simulink model "project_final"  (R2022b)
settings: Solver=VariableStepAuto  StartTime=0.0  StopTime=20  RelTol=1e-3
values from neighbouring files (symbols this model uses):
  A = [0 0 0 1 0 0 0 0 0 0 0 0;     0 0 0 0 1 0 0 0 0 0 0 0;     0 0 0 0 0 1 0 0 0 0 0 0;     0 0 0 0 0 0 0 -g 0 0 0 0;     0 0 0 0 0 0 g 0 0 0 0 0;     0 0 0 0 0 0 0 0 0 0 0 0;     0 0 0 0 0 0 0 0 0 1 0 0;     0 0 0 0 0 0 0 0 0 0 1 0;     0 0 0 0 0 0 0 0 0 0 0 1;     0 0 0 0 0 0 0 0 0 0 0 0;     0 0 0 0 0 0 0 0 0 0 0 0;     0 0 0 0 0 0 0 0 0 0 0 0]    [project_final.m]
  Ax = 0.0    (= 0)    [project_final.m]
  Ay = 0.0    (= 0)    [project_final.m]
  Az = 0.0    (= 0)    [project_final.m]
  B = [0 0 0 0;     0 0 0 0;     0 0 0 0;     0 0 0 0;     0 0 0 0;     1/m 0 0 0;     0 0 0 0;     0 0 0 0;     0 0 0 0;     0 1/Ixx 0 0;     0 0 1/Iyy 0;     0 0 0 1/Izz;]    [project_final.m]
  C = [1 0 0 0 0 0 0 0 0 0 0 0;      0 1 0 0 0 0 0 0 0 0 0 0;      0 0 1 0 0 0 0 0 0 0 0 0;      0 0 0 0 0 0 1 0 0 0 0 0;      0 0 0 0 0 0 0 1 0 0 0 0;      0 0 0 0 0 0 0 0 1 0 0 0;]    [project_final.m]
  D = zeros(6,4)    [project_final.m]
  g = 9.81    [project_final.m]
  Ixx = 0.00963    [project_final.m]
  Iyy = 0.00963    [project_final.m]
  Izz = 0.019    [project_final.m]
  Jr = 5.225e-5    (= 5.225e-05)    [project_final.m]
  l = 0.24    [project_final.m]
  m = 0.82    [project_final.m]
undefined symbols (not defined in the file or in its folder): K_n, K_o, sysK
libraries: simulink x5, simulink_extras x4, visionsinks x2, sim3dcameralib x2, sim3dlib x2, uavsim3dlib x2
settings Model: Creator=isa  LastModifiedBy=Abdullah Ak
settings SolverCC: ZeroCrossAlgorithm=Adaptive
settings DataIOCC: ReturnWorkspaceOutputs=off
settings DebuggingCC: MaskedZcDiagnostic=none  IgnoredZcDiagnostic=none

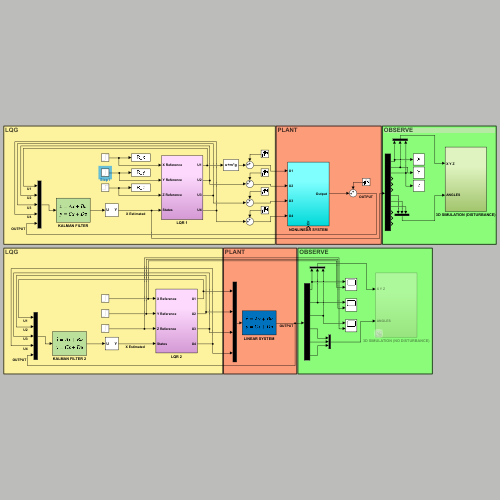
[thumbnail: Simulink's stored preview of the top-level diagram]
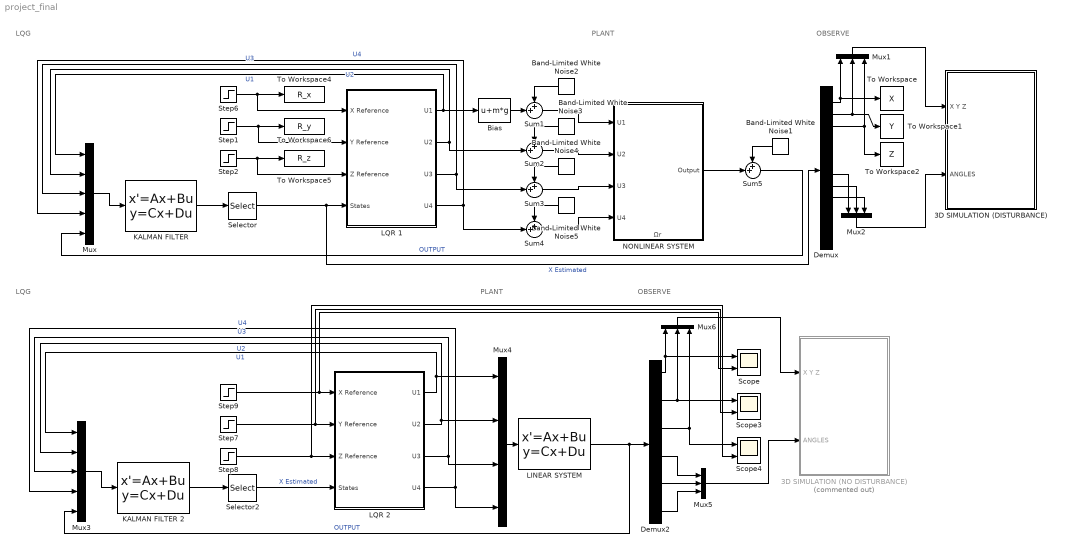
== system project_final ==
  note: OBSERVE
  note: OBSERVE
  note: PLANT
  note: LQG
  note: LQG
  note: PLANT
  3D SIMULATION (DISTURBANCE) : Subsystem
  3D SIMULATION (NO DISTURBANCE) : Subsystem  Commented=on
  Band-Limited White Noise{1..5} (5 alike) : simulink/Sources/Band-Limited White Noise  Cov=[0.0001]  Ts=0.1  seed=[23341]
  Bias : Bias  Bias=m*g  SaturateOnIntegerOverflow=off
  Demux : Demux  Outputs=12
  Demux2 : Demux  Outputs=6
  KALMAN FILTER : StateSpace  A=sysK.A  B=sysK.B  C=sysK.C  D=sysK.D  InitialCondition=0
  KALMAN FILTER 2 : StateSpace  A=sysK.A  B=sysK.B  C=sysK.C  D=sysK.D  InitialCondition=0
  LINEAR SYSTEM : StateSpace  A=A  B=B  C=C  D=D  InitialCondition=0
  LQR 1 : Subsystem
  LQR 2 : Subsystem
  Mux : Mux  Inputs=5
  Mux{1..2,5..6} (4 alike) : Mux  Inputs=3
  Mux3 : Mux  Inputs=5
  Mux4 : Mux
  NONLINEAR SYSTEM : Subsystem
      settings: PortSchema="{\"entries\":[{\"content\":{\"sides\":[{\"content\":{\"connectorIds\":[\"In1\",\"In2\",\"In3\",\"In4\"]},\"type\":\"ConnectorPlacement.EquallySpacedRectSide\",\"uuid\":\"a5503451-5a23-4017-b645-9eb3d3f2dd65\"},{\"content\":{\"connectorIds\":[\"Out1\"],\"side\":\"RIGHT\"},\"type\":\"ConnectorPlacement.EquallySpacedRectSide\",\"uuid\":\"5f9284f0-a452-4177-bce3-aee519bf0d63\"},{\"content\":{\"side\":\"TOP\"},\"type\":\"ConnectorPlacement.EquallySpacedRectSide\",\"uuid\":\"8bc8bc99-887e-4f77-aaa8-21d509049f1f\"},{\"content\":{\"connectorIds\":[\"In5\"],\"side\":\"BOTTOM\"},\"type\":\"ConnectorPlacement.EquallySpacedRectSide\",\"uuid\":\"ae093331-e5e5-4be8-9937-2af24c161ac0\"}]},\"type\":\"ConnectorPlacement.EquallySpacedConnector\",\"uuid\":\"9aea3e95-818c-4bf6-8240-35747b8e2613\"}],\"packageUris\":[\"http://schema.mathworks.com/mf0/Connector/R2020b\"],\"version\":\"1.0\"}"
  Scope : Scope  NumInputPorts=2
  Scope3 : Scope  NumInputPorts=2
  Scope4 : Scope  NumInputPorts=2
  Selector : Selector  InputPortWidth=18  IndexOptions=Index vector (dialog)  Indices=[7:18]  OutputSizes=1
  Selector2 : Selector  InputPortWidth=18  IndexOptions=Index vector (dialog)  Indices=[7:18]  OutputSizes=1
  Step1 : Step  Time=5  After=25  SampleTime=0
  Step2 : Step  After=31  SampleTime=0
  Step6 : Step  Time=10  After=31  SampleTime=0
  Step7 : Step  Time=5  After=8  SampleTime=0
  Step8 : Step  After=10  SampleTime=0
  Step9 : Step  Time=10  After=8  SampleTime=0
  Sum{1..5} (5 alike) : Sum  Inputs=++|
  To Workspace : ToWorkspace  VariableName=X  SaveFormat=Timeseries  SampleTime=-1
  To Workspace1 : ToWorkspace  VariableName=Y  SaveFormat=Timeseries  SampleTime=-1
  To Workspace2 : ToWorkspace  VariableName=Z  SaveFormat=Timeseries  SampleTime=-1
  To Workspace4 : ToWorkspace  VariableName=R_x  SaveFormat=Timeseries  SampleTime=-1
  To Workspace5 : ToWorkspace  VariableName=R_z  SaveFormat=Timeseries  SampleTime=-1
  To Workspace6 : ToWorkspace  VariableName=R_y  SaveFormat=Timeseries  SampleTime=-1
  wires:
  LQR 1/1(U1) -> Bias/1, Mux/1  "U1"
  Bias/1 -> Sum1/2
  LQR 1/2(U2) -> Sum2/2, Mux/2  "U2"
  LQR 1/3(U3) -> Sum3/2, Mux/3  "U3"
  LQR 1/4(U4) -> Sum4/2, Mux/4  "U4"
  KALMAN FILTER/1 -> Selector/1
  Selector/1 -> LQR 1/4(States), Demux/1  "X Estimated"
  Mux/1 -> KALMAN FILTER/1
  Sum5/1 -> Mux/5  "OUTPUT"
  Step1/1 -> LQR 1/2(Y Reference), To Workspace6/1
  Step6/1 -> To Workspace4/1, LQR 1/1(X Reference)
  Step2/1 -> LQR 1/3(Z Reference), To Workspace5/1
  Demux/3 -> To Workspace2/1, Mux1/3
  Demux/1 -> Mux1/1, To Workspace/1
  Demux/2 -> To Workspace1/1, Mux1/2
  Sum1/1 -> NONLINEAR SYSTEM/1(U1)
  Sum2/1 -> NONLINEAR SYSTEM/2(U2)
  Sum3/1 -> NONLINEAR SYSTEM/3(U3)
  Sum4/1 -> NONLINEAR SYSTEM/4(U4)
  NONLINEAR SYSTEM/1("Output ") -> Sum5/2
  Band-Limited White Noise1/1 -> Sum5/1
  Band-Limited White Noise2/1 -> Sum1/1
  Band-Limited White Noise3/1 -> Sum2/1
  Band-Limited White Noise4/1 -> Sum3/1
  Band-Limited White Noise5/1 -> Sum4/1
  Demux2/2 -> Scope3/1, Mux6/2
  Demux2/3 -> Scope4/1, Mux6/3
  Step8/1 -> LQR 2/3(Z Reference), Scope4/2
  Step9/1 -> LQR 2/1(X Reference), Scope/2
  Step7/1 -> LQR 2/2(Y Reference), Scope3/2
  LINEAR SYSTEM/1 -> Mux3/5, Demux2/1  "OUTPUT"
  Mux3/1 -> KALMAN FILTER 2/1
  Selector2/1 -> LQR 2/4(States)  "X Estimated"
  KALMAN FILTER 2/1 -> Selector2/1
  LQR 2/4(U4) -> Mux4/4, Mux3/4  "U4"
  LQR 2/3(U3) -> Mux4/3, Mux3/3  "U3"
  LQR 2/2(U2) -> Mux4/2, Mux3/2  "U2"
  LQR 2/1(U1) -> Mux3/1, Mux4/1  "U1"
  Mux4/1 -> LINEAR SYSTEM/1
  Demux2/1 -> Scope/1, Mux6/1
  Demux2/4 -> Mux5/1
  Demux2/5 -> Mux5/2
  Demux2/6 -> Mux5/3
  Mux6/1 -> 3D SIMULATION (NO DISTURBANCE)/1(X Y Z)
  Mux5/1 -> 3D SIMULATION (NO DISTURBANCE)/2(ANGLES)
  Mux1/1 -> 3D SIMULATION (DISTURBANCE)/1(X Y Z)
  Mux2/1 -> 3D SIMULATION (DISTURBANCE)/2(ANGLES)
  Demux/8 -> Mux2/2
  Demux/9 -> Mux2/3
  Demux/7 -> Mux2/1

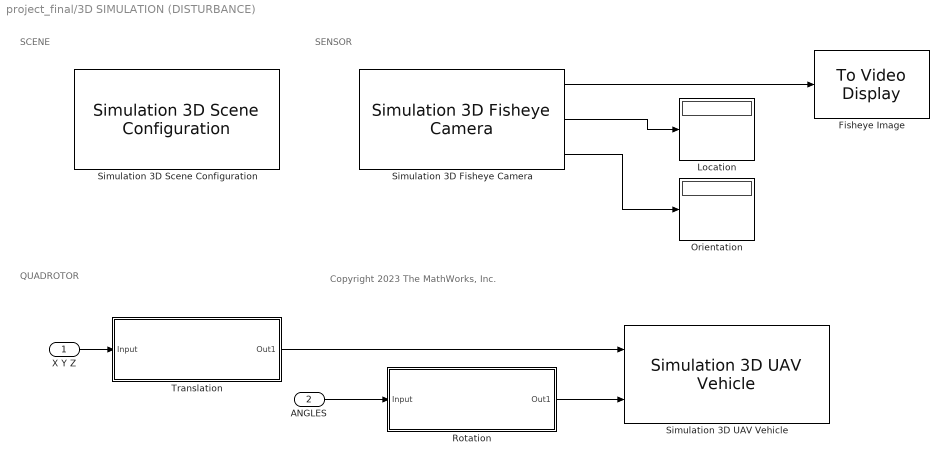
== system project_final/3D SIMULATION (DISTURBANCE) ==
  note: SCENE
  note: QUADROTOR
  note: SENSOR
  note: Copyright 2023 The MathWorks, Inc.
  X Y Z : Inport
  ANGLES : Inport  Port=2
  Fisheye Image : visionsinks/To Video Display  windowSizeMode=Normal  openAtMdlStart=on  fullScreen=off  videoWindowX=2625  videoWindowY=376  saveWindowSize=off  videoWindowWidth=640  videoWindowHeight=640  inputColorFormat=RGB  inputType=Obsolete  imagePorts=One multidimensional signal  OutputDevice=On-screen video monitor  dataOrg=Column-major  isWindowOpen=off
  Location : Display
  Orientation : Display
  Rotation : Subsystem
  Simulation 3D Fisheye Camera : sim3dcameralib/Simulation 3D Fisheye Camera  Priority=1  sensorTag=Sim3dSensor3  sensorId=3  sensorName=Sim3dSensor3  vehTagList={'Q_D';'Scene Origin'}  vehTag=Q_D  mountLoc=Origin  offsetFlag=on  tmountOffset=[0.1, 0, 0]  extTmount=off  rmountOffset=[0, 0, 0]  extRmount=off  OpticalCenter=[640, 360]  ImageSize=[720, 1280]  RadialDistortion=[320, -0.0005, 0, 0]  StretchMatrix=[1, 0; 0, 1]  TransformOutportEnabled=on  SampleTime=-1  mountPoint=[0.1 0 0]  mountOrientation=[0 0 0]  aMode=4  ID=3
  Simulation 3D Scene Configuration : sim3dlib/Simulation 3D Scene Configuration  Priority=0  ProjectFormat=Default Scenes  SceneDesc=US city block  ProjectName=D:\Programlar\MATLAB\R2022B\toolbox\shared\sim3d_projects\automotive_project\UE4\WindowsNoEditor\VehicleSimulation.exe  ScenePath=/Game/Maps/USCityBlock  EnableOpenDRIVE=off  vehTagList={'Q_D';'Scene Origin'}  vehTag=Q_D  OpVisEn=off  Ts=0.3  EnableWindow=on  EnableRemoteAccess=off  EnableWeather=off  SunAltitude=40.0  SunAzimuth=90  clouds=10  wind=0.0  fog=20.0  rain=30  EnableGeospatial=off  OriginHeight=200  OriginLatitude=40.744652  OriginLongitude=-73.988864  MapStyle=Aerial  AdditionalAssetIDs=[]  UseAdvancedSunSky=off  SolarTime=11  TimeZone=-5  Day=21  Month=9  Year=2022  UseDaylightSavingTime=on  DSTStartDay=10  DSTStartMonth=3  DSTEndDay=3  DSTEndMonth=11  DSTSwitchHour=2  sensorTag=MainCamera3  sensorId=3  sensorName=MainCamera3  mountLoc=Origin  offsetFlag=off  tmountOffset=[0, 0, 0]  rmountOffset=[0, 0, 0]  HorizontalResolution=1280  VerticalResolution=720  HorizontalFOV=60  mountPoint=[0 0 0]  mountOrientation=[0 0 0]  aMode=4  ID=3  GeoTrigger=Inactive
  Simulation 3D UAV Vehicle : uavsim3dlib/Simulation 3D UAV Vehicle  Mesh=Quadrotor  MeshPath=/MathWorksUAVContent/UAVs/HexaRotorUAV/HexaRotor.HexaRotor  Color=Black  ActorName=Q_D  InitialTranslation=[0 5 1.5]  InitialRotation=[0 0 0]  SampleTime=-1  ActorType=SimulinkVehicle  ID=C  aMode=4  ActorTag=Q_D
  Translation : Subsystem
  wires:
  Simulation 3D Fisheye Camera/1 -> Fisheye Image/1
  Translation/1(Out1) -> Simulation 3D UAV Vehicle/1
  Simulation 3D Fisheye Camera/3 -> Orientation/1
  X Y Z/1 -> Translation/1(Input)
  ANGLES/1 -> Rotation/1(Input)
  Rotation/1(Out1) -> Simulation 3D UAV Vehicle/2
  Simulation 3D Fisheye Camera/2 -> Location/1

== system project_final/3D SIMULATION (NO DISTURBANCE) ==
  note: SENSOR
  note: QUADROTOR
  note: SCENE
  X Y Z : Inport
  ANGLES : Inport  Port=2
  Fisheye Image : visionsinks/To Video Display  windowSizeMode=Normal  openAtMdlStart=on  fullScreen=off  videoWindowX=2625  videoWindowY=376  saveWindowSize=off  videoWindowWidth=640  videoWindowHeight=640  inputColorFormat=RGB  inputType=Obsolete  imagePorts=One multidimensional signal  OutputDevice=On-screen video monitor  dataOrg=Column-major  isWindowOpen=off
  Location : Display
  Orientation : Display
  Rotation : Subsystem
  Simulation 3D Fisheye Camera : sim3dcameralib/Simulation 3D Fisheye Camera  Priority=1  sensorTag=Sim3dSensor2  sensorId=2  sensorName=Sim3dSensor2  vehTagList={'Q_D';'Q_ND';'Scene Origin'}  vehTag=Q_ND  mountLoc=Origin  offsetFlag=on  tmountOffset=[0.1, 0, 0]  extTmount=off  rmountOffset=[0, 0, 0]  extRmount=off  OpticalCenter=[640, 360]  ImageSize=[720, 1280]  RadialDistortion=[320, -0.0005, 0, 0]  StretchMatrix=[1, 0; 0, 1]  TransformOutportEnabled=on  SampleTime=-1  mountPoint=[0.1 0 0]  mountOrientation=[0 0 0]  aMode=4  ID=2
  Simulation 3D Scene Configuration : sim3dlib/Simulation 3D Scene Configuration  Priority=0  ProjectFormat=Default Scenes  SceneDesc=US city block  ProjectName=D:\Programlar\MATLAB\R2022B\toolbox\shared\sim3d_projects\automotive_project\UE4\WindowsNoEditor\VehicleSimulation.exe  ScenePath=/Game/Maps/USCityBlock  EnableOpenDRIVE=off  vehTagList={'Q_D';'Q_ND';'Scene Origin'}  vehTag=Q_ND  OpVisEn=off  Ts=0.3  EnableWindow=on  EnableRemoteAccess=off  EnableWeather=off  SunAltitude=40.0  SunAzimuth=90  clouds=10  wind=1  fog=0  rain=0  EnableGeospatial=off  OriginHeight=200  OriginLatitude=40.744652  OriginLongitude=-73.988864  MapStyle=Aerial  AdditionalAssetIDs=[]  UseAdvancedSunSky=off  SolarTime=11  TimeZone=-5  Day=21  Month=9  Year=2022  UseDaylightSavingTime=on  DSTStartDay=10  DSTStartMonth=3  DSTEndDay=3  DSTEndMonth=11  DSTSwitchHour=2  sensorTag=MainCamera2  sensorId=2  sensorName=MainCamera2  mountLoc=Origin  offsetFlag=off  tmountOffset=[0, 0, 0]  rmountOffset=[0, 0, 0]  HorizontalResolution=1280  VerticalResolution=720  HorizontalFOV=60  mountPoint=[0 0 0]  mountOrientation=[0 0 0]  aMode=4  ID=2  GeoTrigger=Inactive
  Simulation 3D UAV Vehicle : uavsim3dlib/Simulation 3D UAV Vehicle  Mesh=Quadrotor  MeshPath=/MathWorksUAVContent/UAVs/HexaRotorUAV/HexaRotor.HexaRotor  Color=White  ActorName=Q_ND  InitialTranslation=[0 5 1.5]  InitialRotation=[0 0 0]  SampleTime=-1  ActorType=SimulinkVehicle  ID=C  aMode=4  ActorTag=Q_ND
  Translation : Subsystem
  wires:
  Simulation 3D Fisheye Camera/2 -> Location/1
  Rotation/1(Out1) -> Simulation 3D UAV Vehicle/2
  ANGLES/1 -> Rotation/1(Input)
  X Y Z/1 -> Translation/1(Input)
  Simulation 3D Fisheye Camera/3 -> Orientation/1
  Translation/1(Out1) -> Simulation 3D UAV Vehicle/1
  Simulation 3D Fisheye Camera/1 -> Fisheye Image/1

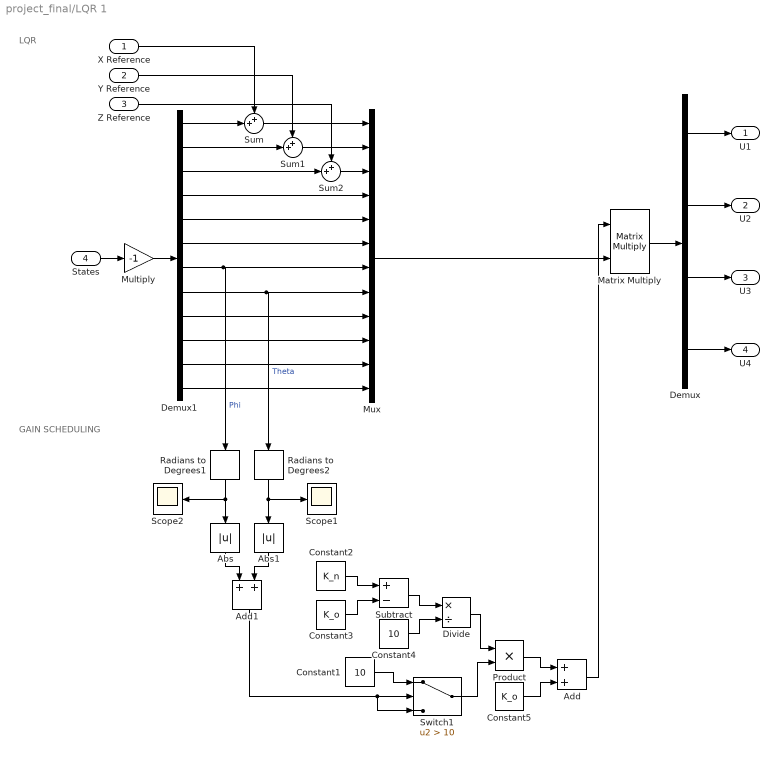
== system project_final/LQR 1 ==
  note: GAIN SCHEDULING
  note: LQR
  X Reference : Inport
  Y Reference : Inport  Port=2
  Z Reference : Inport  Port=3
  States : Inport  Port=4
  Abs : Abs  SaturateOnIntegerOverflow=off
  Abs1 : Abs  SaturateOnIntegerOverflow=off
  Add : Sum
  Add1 : Sum
  Constant1 : Constant  Value=10
  Constant2 : Constant  Value=K_n
  Constant3 : Constant  Value=K_o
  Constant4 : Constant  Value=10
  Constant5 : Constant  Value=K_o
  Demux : Demux
  Demux1 : Demux  Outputs=12
  Divide : Product  Inputs=*/
  Matrix Multiply : Product  Multiplication=Matrix(*)
  Multiply : Gain  Gain=-1
  Mux : Mux  Inputs=12
  Product : Product
  Radians to Degrees1 : simulink_extras/Transformations/Radians to Degrees
  Radians to Degrees2 : simulink_extras/Transformations/Radians to Degrees
  Scope1 : Scope
  Scope2 : Scope
  Subtract : Sum  Inputs=+-
  Sum : Sum  Inputs=++|
  Sum1 : Sum  Inputs=++|
  Sum2 : Sum  Inputs=++|
  Switch1 : Switch  Criteria=u2 > Threshold  Threshold=10  SaturateOnIntegerOverflow=off  InputSameDT=off
  U1 : Outport
  U2 : Outport  Port=2
  U3 : Outport  Port=3
  U4 : Outport  Port=4
  wires:
  Matrix Multiply/1 -> Demux/1
  Demux/1 -> U1/1
  Demux/2 -> U2/1
  Demux/3 -> U3/1
  Demux/4 -> U4/1
  Z Reference/1 -> Sum2/1
  X Reference/1 -> Sum/1
  Y Reference/1 -> Sum1/1
  States/1 -> Multiply/1
  Demux1/1 -> Sum/2
  Demux1/2 -> Sum1/2
  Demux1/3 -> Sum2/2
  Sum/1 -> Mux/1
  Sum1/1 -> Mux/2
  Sum2/1 -> Mux/3
  Demux1/4 -> Mux/4
  Demux1/5 -> Mux/5
  Demux1/6 -> Mux/6
  Demux1/7 -> Mux/7, Radians to Degrees1/1  "Phi"
  Demux1/8 -> Mux/8, Radians to Degrees2/1  "Theta"
  Demux1/9 -> Mux/9
  Demux1/10 -> Mux/10
  Demux1/12 -> Mux/12
  Mux/1 -> Matrix Multiply/2
  Multiply/1 -> Demux1/1
  Constant1/1 -> Switch1/1
  Constant3/1 -> Subtract/2
  Constant2/1 -> Subtract/1
  Subtract/1 -> Divide/1
  Constant4/1 -> Divide/2
  Divide/1 -> Product/1
  Switch1/1 -> Product/2
  Product/1 -> Add/1
  Constant5/1 -> Add/2
  Add/1 -> Matrix Multiply/1
  Radians to Degrees2/1 -> Scope1/1, Abs1/1
  Radians to Degrees1/1 -> Scope2/1, Abs/1
  Abs1/1 -> Add1/2
  Abs/1 -> Add1/1
  Add1/1 -> Switch1/3, Switch1/2
  Demux1/11 -> Mux/11

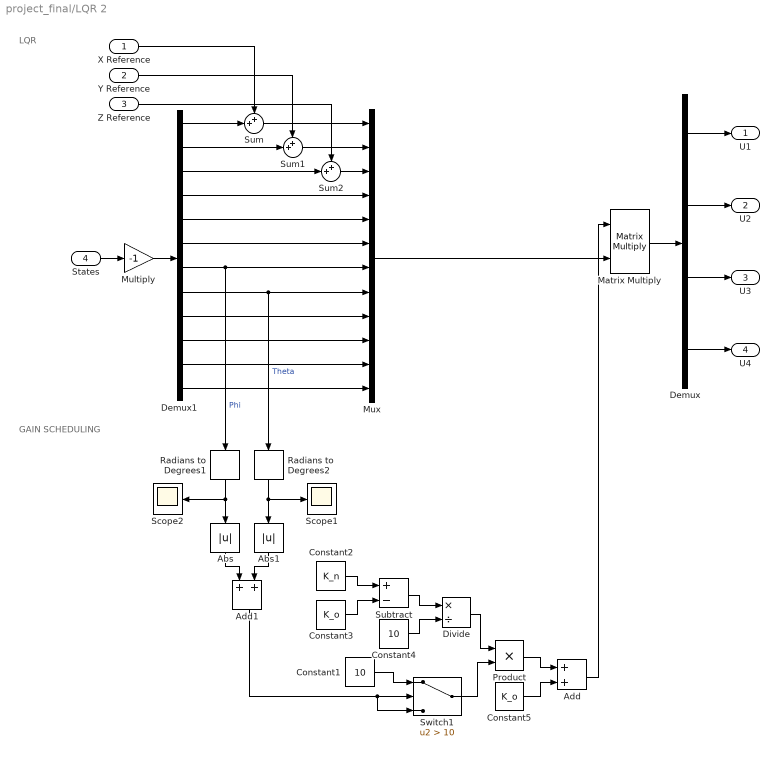
== system project_final/LQR 2 ==
  note: LQR
  note: GAIN SCHEDULING
  X Reference : Inport
  Y Reference : Inport  Port=2
  Z Reference : Inport  Port=3
  States : Inport  Port=4
  Abs : Abs  SaturateOnIntegerOverflow=off
  Abs1 : Abs  SaturateOnIntegerOverflow=off
  Add : Sum
  Add1 : Sum
  Constant1 : Constant  Value=10
  Constant2 : Constant  Value=K_n
  Constant3 : Constant  Value=K_o
  Constant4 : Constant  Value=10
  Constant5 : Constant  Value=K_o
  Demux : Demux
  Demux1 : Demux  Outputs=12
  Divide : Product  Inputs=*/
  Matrix Multiply : Product  Multiplication=Matrix(*)
  Multiply : Gain  Gain=-1
  Mux : Mux  Inputs=12
  Product : Product
  Radians to Degrees1 : simulink_extras/Transformations/Radians to Degrees
  Radians to Degrees2 : simulink_extras/Transformations/Radians to Degrees
  Scope1 : Scope
  Scope2 : Scope
  Subtract : Sum  Inputs=+-
  Sum : Sum  Inputs=++|
  Sum1 : Sum  Inputs=++|
  Sum2 : Sum  Inputs=++|
  Switch1 : Switch  Criteria=u2 > Threshold  Threshold=10  SaturateOnIntegerOverflow=off  InputSameDT=off
  U1 : Outport
  U2 : Outport  Port=2
  U3 : Outport  Port=3
  U4 : Outport  Port=4
  wires:
  Demux1/7 -> Mux/7, Radians to Degrees1/1  "Phi"
  Abs/1 -> Add1/1
  Demux1/11 -> Mux/11
  Subtract/1 -> Divide/1
  Demux1/10 -> Mux/10
  Add/1 -> Matrix Multiply/1
  Demux1/1 -> Sum/2
  Radians to Degrees1/1 -> Scope2/1, Abs/1
  Constant4/1 -> Divide/2
  Constant5/1 -> Add/2
  Demux/4 -> U4/1
  Product/1 -> Add/1
  Demux/3 -> U3/1
  Demux/2 -> U2/1
  Demux1/4 -> Mux/4
  Switch1/1 -> Product/2
  Radians to Degrees2/1 -> Scope1/1, Abs1/1
  States/1 -> Multiply/1
  Demux1/12 -> Mux/12
  Demux/1 -> U1/1
  Constant3/1 -> Subtract/2
  Demux1/8 -> Mux/8, Radians to Degrees2/1  "Theta"
  Demux1/5 -> Mux/5
  Constant1/1 -> Switch1/1
  Sum/1 -> Mux/1
  Demux1/9 -> Mux/9
  Abs1/1 -> Add1/2
  Sum2/1 -> Mux/3
  Constant2/1 -> Subtract/1
  X Reference/1 -> Sum/1
  Sum1/1 -> Mux/2
  Demux1/2 -> Sum1/2
  Y Reference/1 -> Sum1/1
  Demux1/3 -> Sum2/2
  Mux/1 -> Matrix Multiply/2
  Matrix Multiply/1 -> Demux/1
  Divide/1 -> Product/1
  Z Reference/1 -> Sum2/1
  Demux1/6 -> Mux/6
  Add1/1 -> Switch1/3, Switch1/2
  Multiply/1 -> Demux1/1

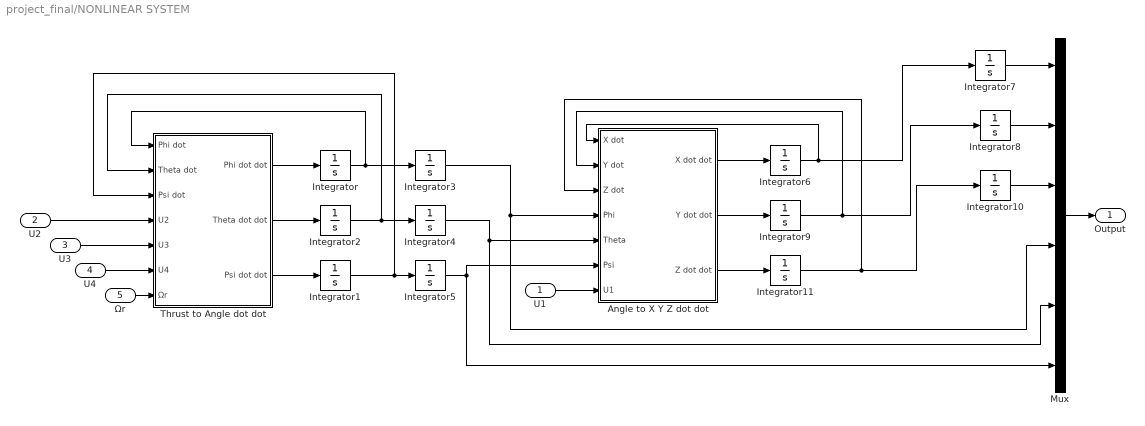
== system project_final/NONLINEAR SYSTEM ==
  U1 : Inport
  U2 : Inport  Port=2
  U3 : Inport  Port=3
  U4 : Inport  Port=4
  Ωr : Inport  Port=5
  Angle to X Y Z dot dot : Subsystem
  Integrator{,1..2,6..9,11} (8 alike) : Integrator
  Integrator10 : Integrator  LimitOutput=on  LowerSaturationLimit=0
  Integrator3 : Integrator  WrapState=on
  Integrator4 : Integrator  UpperSaturationLimit=pi  LowerSaturationLimit=-pi  WrapState=on
  Integrator5 : Integrator  WrapState=on
  Mux : Mux  Inputs=6
  Thrust to Angle dot dot : Subsystem
  "Output " : Outport
  wires:
  Thrust to Angle dot dot/1(Phi dot dot) -> Integrator/1
  Integrator/1 -> Integrator3/1, Thrust to Angle dot dot/1(Phi dot)
  Thrust to Angle dot dot/2(Theta dot dot) -> Integrator2/1
  Thrust to Angle dot dot/3(Psi dot dot) -> Integrator1/1
  Integrator2/1 -> Integrator4/1, Thrust to Angle dot dot/2(Theta dot)
  Integrator1/1 -> Integrator5/1, Thrust to Angle dot dot/3(Psi dot)
  Integrator5/1 -> Angle to X Y Z dot dot/6(Psi), Mux/6
  Integrator4/1 -> Angle to X Y Z dot dot/5(Theta), Mux/5
  Integrator3/1 -> Angle to X Y Z dot dot/4(Phi), Mux/4
  Angle to X Y Z dot dot/3(Z dot dot) -> Integrator11/1
  Angle to X Y Z dot dot/2(Y dot dot) -> Integrator9/1
  Angle to X Y Z dot dot/1(X dot dot) -> Integrator6/1
  Integrator6/1 -> Angle to X Y Z dot dot/1(X dot), Integrator7/1
  Integrator9/1 -> Angle to X Y Z dot dot/2(Y dot), Integrator8/1
  Integrator11/1 -> Integrator10/1, Angle to X Y Z dot dot/3(Z dot)
  U2/1 -> Thrust to Angle dot dot/4(U2)
  U3/1 -> Thrust to Angle dot dot/5(U3)
  U4/1 -> Thrust to Angle dot dot/6(U4)
  Ωr/1 -> Thrust to Angle dot dot/7(Ωr)
  U1/1 -> Angle to X Y Z dot dot/7(U1)
  Integrator7/1 -> Mux/1
  Integrator8/1 -> Mux/2
  Integrator10/1 -> Mux/3
  Mux/1 -> "Output "/1

== system project_final/3D SIMULATION (DISTURBANCE)/Rotation ==
  Input : Inport
  Demux : Demux  Outputs=3
  Mux : Mux  Inputs=3
  Out1 : Outport
  wires:
  Mux/1 -> Out1/1
  Input/1 -> Demux/1
  Demux/1 -> Mux/1
  Demux/2 -> Mux/2
  Demux/3 -> Mux/3

== system project_final/3D SIMULATION (DISTURBANCE)/Translation ==
  Input : Inport
  Demux : Demux  Outputs=3
  Mux : Mux  Inputs=3
  Out1 : Outport
  wires:
  Mux/1 -> Out1/1
  Demux/1 -> Mux/1
  Demux/2 -> Mux/2
  Demux/3 -> Mux/3
  Input/1 -> Demux/1

== system project_final/3D SIMULATION (NO DISTURBANCE)/Rotation ==
  Input : Inport
  Demux : Demux  Outputs=3
  Mux : Mux  Inputs=3
  Out1 : Outport
  wires:
  Demux/3 -> Mux/3
  Demux/2 -> Mux/2
  Demux/1 -> Mux/1
  Input/1 -> Demux/1
  Mux/1 -> Out1/1

== system project_final/3D SIMULATION (NO DISTURBANCE)/Translation ==
  Input : Inport
  Demux : Demux  Outputs=3
  Mux : Mux  Inputs=3
  Out1 : Outport
  wires:
  Input/1 -> Demux/1
  Demux/3 -> Mux/3
  Demux/2 -> Mux/2
  Demux/1 -> Mux/1
  Mux/1 -> Out1/1

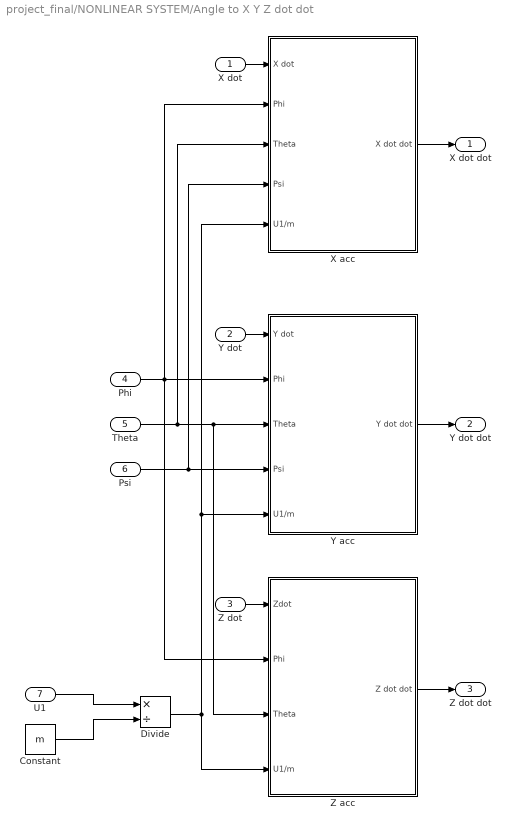
== system project_final/NONLINEAR SYSTEM/Angle to X Y Z dot dot ==
  X dot : Inport
  Y dot : Inport  Port=2
  Z dot : Inport  Port=3
  Phi : Inport  Port=4
  Theta : Inport  Port=5
  Psi : Inport  Port=6
  U1 : Inport  Port=7
  Constant : Constant  Value=m
  Divide : Product  Inputs=*/
  X acc : Subsystem
  Y acc : Subsystem
  Z acc : Subsystem
  X dot dot : Outport
  Y dot dot : Outport  Port=2
  Z dot dot : Outport  Port=3
  wires:
  X acc/1(X dot dot) -> X dot dot/1
  Y acc/1(Y dot dot) -> Y dot dot/1
  Z acc/1(Z dot dot) -> Z dot dot/1
  U1/1 -> Divide/1
  Constant/1 -> Divide/2
  Divide/1 -> Z acc/4(U1/m), Y acc/5(U1/m), X acc/5(U1/m)
  X dot/1 -> X acc/1(X dot)
  Y dot/1 -> Y acc/1(Y dot)
  Z dot/1 -> Z acc/1(Zdot)
  Theta/1 -> Y acc/3(Theta), Z acc/3(Theta), X acc/3(Theta)
  Phi/1 -> Y acc/2(Phi), Z acc/2(Phi), X acc/2(Phi)
  Psi/1 -> Y acc/4(Psi), X acc/4(Psi)

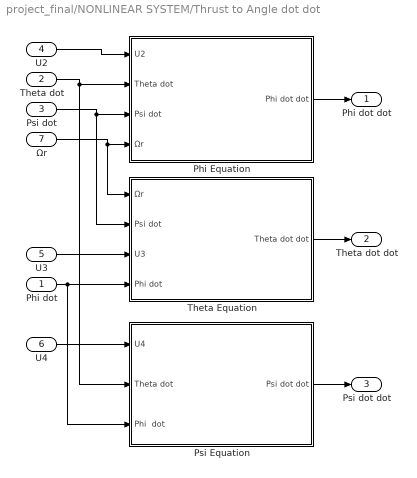
== system project_final/NONLINEAR SYSTEM/Thrust to Angle dot dot ==
  Phi dot : Inport
  Theta dot : Inport  Port=2
  Psi dot : Inport  Port=3
  U2 : Inport  Port=4
  U3 : Inport  Port=5
  U4 : Inport  Port=6
  Ωr : Inport  Port=7
  Phi Equation : Subsystem
  Psi Equation : Subsystem
  Theta Equation : Subsystem
  Phi dot dot : Outport
  Theta dot dot : Outport  Port=2
  Psi dot dot : Outport  Port=3
  wires:
  Ωr/1 -> Theta Equation/1(Ωr), Phi Equation/4(Ωr)
  Psi dot/1 -> Theta Equation/2(Psi dot), Phi Equation/3(Psi dot)
  Theta dot/1 -> Psi Equation/2(Theta dot), Phi Equation/2(Theta dot)
  U2/1 -> Phi Equation/1(U2)
  Phi Equation/1(Phi dot dot) -> Phi dot dot/1
  Psi Equation/1(Psi dot dot) -> Psi dot dot/1
  U3/1 -> Theta Equation/3(U3)
  Phi dot/1 -> Theta Equation/4(Phi dot), Psi Equation/3(Phi  dot)
  U4/1 -> Psi Equation/1(U4)
  Theta Equation/1(Theta dot dot) -> Theta dot dot/1

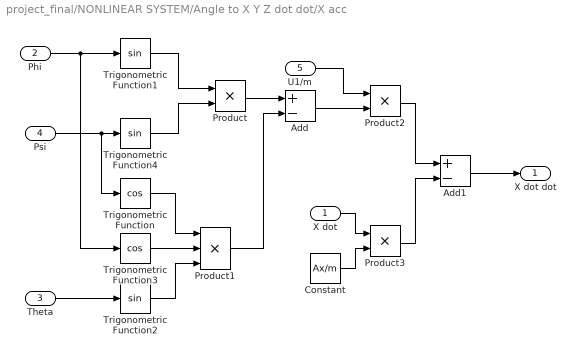
== system project_final/NONLINEAR SYSTEM/Angle to X Y Z dot dot/X acc ==
  X dot : Inport
  Phi : Inport  Port=2
  Theta : Inport  Port=3
  Psi : Inport  Port=4
  U1/m : Inport  Port=5
  Add : Sum  Inputs=+-
  Add1 : Sum  Inputs=+-
  Constant : Constant  Value=Ax/m
  Product : Product
  Product1 : Product  Inputs=3
  Product2 : Product
  Product3 : Product
  Trigonometric Function : Trigonometry  Operator=cos
  Trigonometric Function1 : Trigonometry
  Trigonometric Function2 : Trigonometry
  Trigonometric Function3 : Trigonometry  Operator=cos
  Trigonometric Function4 : Trigonometry
  X dot dot : Outport
  wires:
  Psi/1 -> Trigonometric Function/1, Trigonometric Function4/1
  Trigonometric Function4/1 -> Product/2
  Phi/1 -> Trigonometric Function3/1, Trigonometric Function1/1
  Trigonometric Function3/1 -> Product1/2
  Trigonometric Function1/1 -> Product/1
  Theta/1 -> Trigonometric Function2/1
  Product/1 -> Add/1
  Trigonometric Function/1 -> Product1/1
  Trigonometric Function2/1 -> Product1/3
  Product1/1 -> Add/2
  Add/1 -> Product2/2
  U1/m/1 -> Product2/1
  Product2/1 -> Add1/1
  X dot/1 -> Product3/1
  Constant/1 -> Product3/2
  Product3/1 -> Add1/2
  Add1/1 -> X dot dot/1

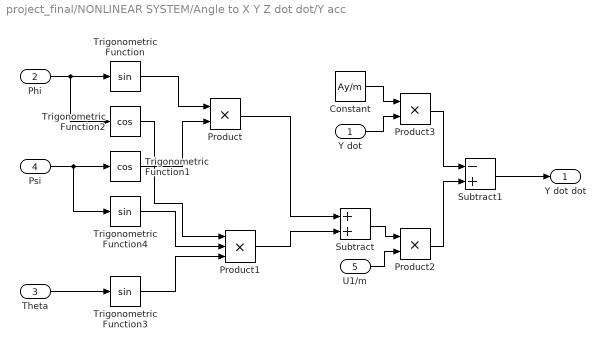
== system project_final/NONLINEAR SYSTEM/Angle to X Y Z dot dot/Y acc ==
  Y dot : Inport
  Phi : Inport  Port=2
  Theta : Inport  Port=3
  Psi : Inport  Port=4
  U1/m : Inport  Port=5
  Constant : Constant  Value=Ay/m
  Product : Product
  Product1 : Product  Inputs=3
  Product2 : Product
  Product3 : Product
  Subtract : Sum
  Subtract1 : Sum  Inputs=-+
  Trigonometric Function : Trigonometry
  Trigonometric Function1 : Trigonometry  Operator=cos
  Trigonometric Function2 : Trigonometry  Operator=cos
  Trigonometric Function3 : Trigonometry
  Trigonometric Function4 : Trigonometry
  Y dot dot : Outport
  wires:
  Psi/1 -> Trigonometric Function4/1, Trigonometric Function1/1
  Phi/1 -> Trigonometric Function2/1, Trigonometric Function/1
  Trigonometric Function/1 -> Product/1
  Trigonometric Function1/1 -> Product/2
  Product/1 -> Subtract/1
  Theta/1 -> Trigonometric Function3/1
  Trigonometric Function2/1 -> Product1/1
  Trigonometric Function4/1 -> Product1/2
  Trigonometric Function3/1 -> Product1/3
  Product1/1 -> Subtract/2
  U1/m/1 -> Product2/2
  Subtract/1 -> Product2/1
  Constant/1 -> Product3/1
  Y dot/1 -> Product3/2
  Product3/1 -> Subtract1/1
  Product2/1 -> Subtract1/2
  Subtract1/1 -> Y dot dot/1

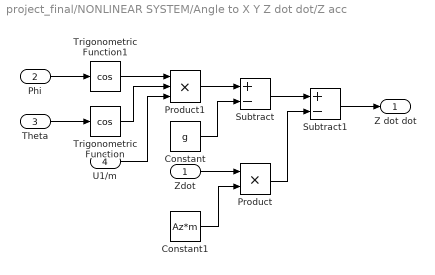
== system project_final/NONLINEAR SYSTEM/Angle to X Y Z dot dot/Z acc ==
  Zdot : Inport
  Phi : Inport  Port=2
  Theta : Inport  Port=3
  U1/m : Inport  Port=4
  Constant : Constant  Value=g
  Constant1 : Constant  Value=Az*m
  Product : Product
  Product1 : Product  Inputs=3
  Subtract : Sum  Inputs=+-
  Subtract1 : Sum  Inputs=+-
  Trigonometric Function : Trigonometry  Operator=cos
  Trigonometric Function1 : Trigonometry  Operator=cos
  Z dot dot : Outport
  wires:
  Phi/1 -> Trigonometric Function1/1
  Theta/1 -> Trigonometric Function/1
  Zdot/1 -> Product/1
  Product1/1 -> Subtract/1
  Trigonometric Function1/1 -> Product1/1
  Trigonometric Function/1 -> Product1/2
  U1/m/1 -> Product1/3
  Constant/1 -> Subtract/2
  Constant1/1 -> Product/2
  Subtract/1 -> Subtract1/1
  Product/1 -> Subtract1/2
  Subtract1/1 -> Z dot dot/1

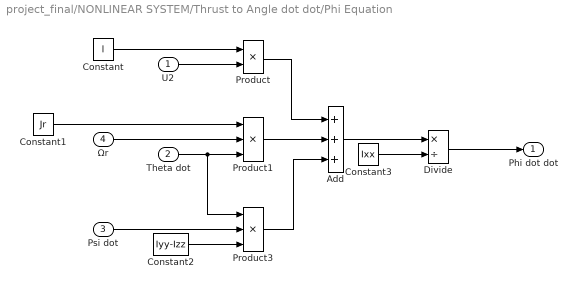
== system project_final/NONLINEAR SYSTEM/Thrust to Angle dot dot/Phi Equation ==
  U2 : Inport
  Theta dot : Inport  Port=2
  Psi dot : Inport  Port=3
  Ωr : Inport  Port=4
  Add : Sum  Inputs=+++
  Constant : Constant  Value=l
  Constant1 : Constant  Value=Jr
  Constant2 : Constant  Value=Iyy-Izz
  Constant3 : Constant  Value=Ixx
  Divide : Product  Inputs=*/
  Product : Product
  Product1 : Product  Inputs=3
  Product3 : Product  Inputs=3
  Phi dot dot : Outport
  wires:
  Ωr/1 -> Product1/2
  Constant/1 -> Product/1
  U2/1 -> Product/2
  Constant1/1 -> Product1/1
  Theta dot/1 -> Product3/1, Product1/3
  Psi dot/1 -> Product3/2
  Product/1 -> Add/1
  Product3/1 -> Add/3
  Constant2/1 -> Product3/3
  Product1/1 -> Add/2
  Add/1 -> Divide/1
  Constant3/1 -> Divide/2
  Divide/1 -> Phi dot dot/1

== system project_final/NONLINEAR SYSTEM/Thrust to Angle dot dot/Psi Equation ==
  U4 : Inport
  Theta dot : Inport  Port=2
  Phi  dot : Inport  Port=3
  Add : Sum
  Constant : Constant  Value=Ixx-Iyy
  Constant1 : Constant  Value=Izz
  Divide : Product  Inputs=*/
  Product : Product  Inputs=3
  Psi dot dot : Outport
  wires:
  Constant/1 -> Product/1
  Theta dot/1 -> Product/2
  Phi  dot/1 -> Product/3
  Product/1 -> Add/2
  U4/1 -> Add/1
  Add/1 -> Divide/1
  Constant1/1 -> Divide/2
  Divide/1 -> Psi dot dot/1

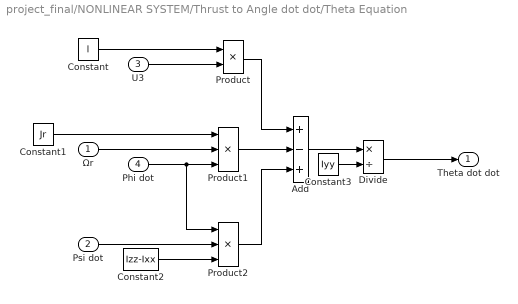
== system project_final/NONLINEAR SYSTEM/Thrust to Angle dot dot/Theta Equation ==
  Ωr : Inport
  Psi dot : Inport  Port=2
  U3 : Inport  Port=3
  Phi dot : Inport  Port=4
  Add : Sum  Inputs=+-+
  Constant : Constant  Value=l
  Constant1 : Constant  Value=Jr
  Constant2 : Constant  Value=Izz-Ixx
  Constant3 : Constant  Value=Iyy
  Divide : Product  Inputs=*/
  Product : Product
  Product1 : Product  Inputs=3
  Product2 : Product  Inputs=3
  Theta dot dot : Outport
  wires:
  Ωr/1 -> Product1/2
  Constant1/1 -> Product1/1
  Constant/1 -> Product/1
  Constant2/1 -> Product2/3
  U3/1 -> Product/2
  Phi dot/1 -> Product1/3, Product2/1
  Psi dot/1 -> Product2/2
  Product/1 -> Add/1
  Product1/1 -> Add/2
  Product2/1 -> Add/3
  Constant3/1 -> Divide/2
  Divide/1 -> Theta dot dot/1
  Add/1 -> Divide/1
